simulink model "SistEqLTI"  (R2023b)
settings: Solver=VariableStepAuto  StartTime=0.0  StopTime=10.0  RelTol=1e-3
values from neighbouring files (symbols this model uses):
  b_eq = b_m + b_l/(r^2)    (= 2.19444444444e-05)    [Parametros.m]
  C_ts = 0.818    [Parametros.m]
  g = 9.80665    [Parametros.m]
  J_eq = J_m + J_l/(r^2)    [Parametros.m]
  k_l = m*l_cm + m_l(1)*l_l    [Parametros.m]
  L_q = 5.8E-3    (= 0.0058)    [Parametros.m]
  lambda_m = 0.016    [Parametros.m]
  P_p = 3    [Parametros.m]
  r = 120    [Parametros.m]
  R_tsamb = 146.7    [Parametros.m]
  Rs_ref = 1.02    [Parametros.m]
settings Model: Creator=Tomas  LastModifiedBy=matia
settings DebuggingCC: UnconnectedInputMsg=warning  UnconnectedOutputMsg=warning  UnconnectedLineMsg=warning
settings ModelReferenceCC: EnableRefExpFcnMdlSchedulingChecks=on
settings RTWCC: DLArmComputeVersion=19.05

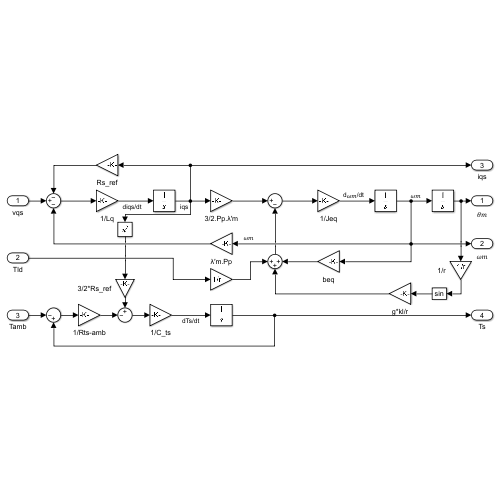
[thumbnail: Simulink's stored preview of the top-level diagram]
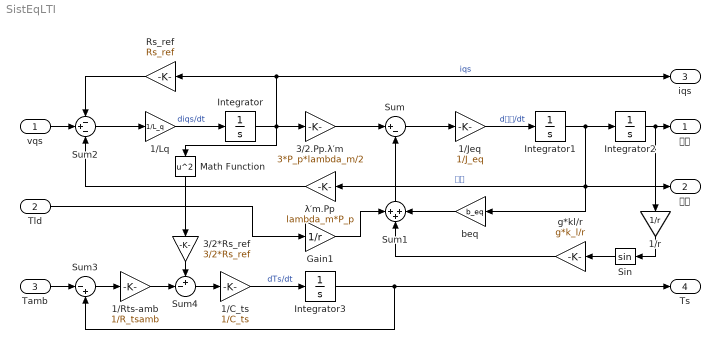
== system SistEqLTI ==
  vqs : Inport
  Tld : Inport  Port=2
  Tamb : Inport  Port=3
  1/C_ts : Gain  Gain=1/C_ts
  1/Jeq : Gain  Gain=1/J_eq
  1/Lq : Gain  Gain=1/L_q
  1/Rts-amb : Gain  Gain=1/R_tsamb
  1/r : Gain  Gain=1/r
  3/2*Rs_ref : Gain  Gain=3/2*Rs_ref
  3/2.Pp.λ′m : Gain  Gain=3*P_p*lambda_m/2
  Gain1 : Gain  Gain=1/r
  Integrator{,1..3} (4 alike) : Integrator
  Math Function : Math  Operator=square
  Rs_ref : Gain  Gain=Rs_ref
  Sin : Trigonometry
  Sum : Sum  Inputs=|+-
  Sum1 : Sum  Inputs=+++
  Sum2 : Sum  Inputs=-+-
  Sum3 : Sum  Inputs=|-+
  Sum4 : Sum  Inputs=+-|
  beq : Gain  Gain=b_eq
  g*kl/r : Gain  Gain=g*k_l/r
  λ′m.Pp : Gain  Gain=lambda_m*P_p
  𝜃𝑚 : Outport
  𝜔𝑚 : Outport  Port=2
  iqs : Outport  Port=3
  Ts : Outport  Port=4
  wires:
  Sum/1 -> 1/Jeq/1
  Sum1/1 -> Sum/2
  Tld/1 -> Gain1/1
  Integrator2/1 -> 1/r/1, 𝜃𝑚/1
  Integrator1/1 -> Integrator2/1, λ′m.Pp/1, beq/1, 𝜔𝑚/1  "𝜔𝑚"
  1/Jeq/1 -> Integrator1/1  "d𝜔𝑚/dt"
  1/Lq/1 -> Integrator/1  "diqs/dt"
  Integrator/1 -> 3/2.Pp.λ′m/1, Math Function/1, Rs_ref/1, iqs/1  "iqs"
  Sum2/1 -> 1/Lq/1
  λ′m.Pp/1 -> Sum2/3
  vqs/1 -> Sum2/2
  Rs_ref/1 -> Sum2/1
  Sum3/1 -> 1/Rts-amb/1
  1/Rts-amb/1 -> Sum4/2
  Math Function/1 -> 3/2*Rs_ref/1
  3/2*Rs_ref/1 -> Sum4/1
  Sum4/1 -> 1/C_ts/1
  1/C_ts/1 -> Integrator3/1  "dTs/dt"
  Tamb/1 -> Sum3/1
  Integrator3/1 -> Sum3/2, Ts/1
  1/r/1 -> Sin/1
  Sin/1 -> g*kl/r/1
  3/2.Pp.λ′m/1 -> Sum/1
  beq/1 -> Sum1/3
  g*kl/r/1 -> Sum1/2
  Gain1/1 -> Sum1/1
